simulink model "automata"  (R2020b)
settings: Solver=VariableStepAuto  StartTime=0.0  StopTime=100  RelTol=1e-3
model workspace (MAT data in the model file):
  G_sup_tsp = Simulink.Signal
  G_sup_tsp.DataType = 'double'
  G_sup_tsp.Dimensions = -1
  G_sup_tsp.DimensionsMode = 'auto'
  G_sup_tsp.Complexity = 'real'
  G_sup_tsp.SampleTime = -1
  G_sup_tsp.SamplingMode = 'auto'
  G_sup_tsp.InitialValue = '175'
  G_sup_tsp_ideal = Simulink.Signal
  G_sup_tsp_ideal.DataType = 'double'
  G_sup_tsp_ideal.Dimensions = -1
  G_sup_tsp_ideal.DimensionsMode = 'auto'
  G_sup_tsp_ideal.Complexity = 'real'
  G_sup_tsp_ideal.SampleTime = -1
  G_sup_tsp_ideal.SamplingMode = 'auto'
  G_sup_tsp_ideal.InitialValue = '175'
  G_sup_tsp_noneAct = Simulink.Signal
  G_sup_tsp_noneAct.DataType = 'double'
  G_sup_tsp_noneAct.Dimensions = -1
  G_sup_tsp_noneAct.DimensionsMode = 'auto'
  G_sup_tsp_noneAct.Complexity = 'real'
  G_sup_tsp_noneAct.SampleTime = -1
  G_sup_tsp_noneAct.SamplingMode = 'auto'
  G_sup_tsp_noneAct.InitialValue = '175'
undefined symbols (not defined in the file): WLAN
libraries: truetime x3, pid_lib x2, simulink x1
settings Model: Creator=Mr_Li  LastModifiedBy=Mr_Li

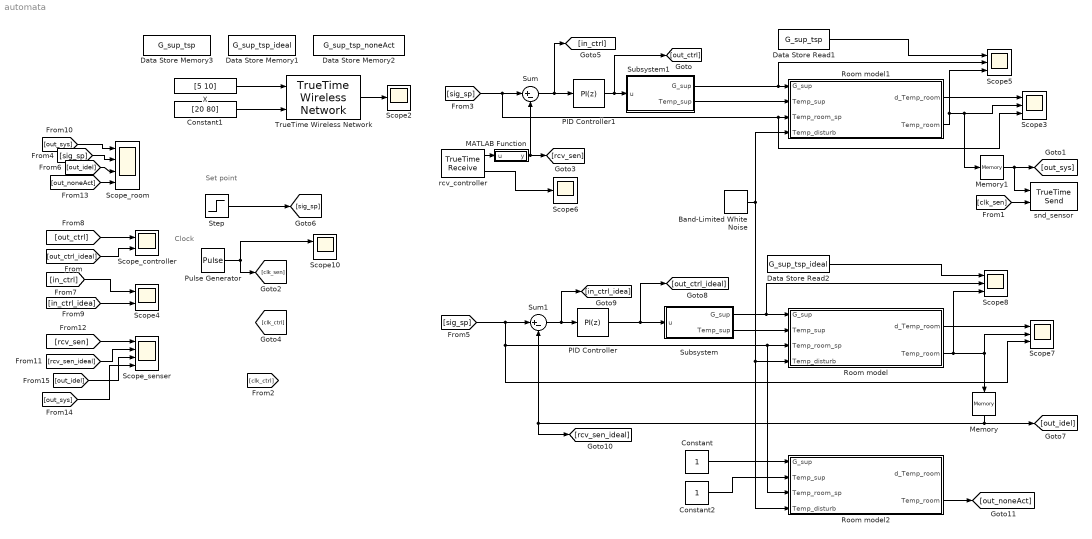
== system automata ==
  note: Set point
  note: Clock
  Band-Limited White Noise : simulink/Sources/Band-Limited White Noise  Cov=[0.01]  Ts=1  seed=[23341]
  Constant : Constant
  Constant1 : Constant  Value=[20 80]  VectorParams1D=off
  Constant2 : Constant
  Data Store Memory1 : DataStoreMemory  DataStoreName=G_sup_tsp_ideal  ReadBeforeWriteMsg=warning  WriteAfterWriteMsg=warning  WriteAfterReadMsg=warning  InitialValue=175  ShowAdditionalParam=off  OutDataTypeStr=double
  Data Store Memory2 : DataStoreMemory  DataStoreName=G_sup_tsp_noneAct  ReadBeforeWriteMsg=warning  WriteAfterWriteMsg=warning  WriteAfterReadMsg=warning  InitialValue=175  ShowAdditionalParam=off  OutDataTypeStr=double
  Data Store Memory3 : DataStoreMemory  DataStoreName=G_sup_tsp  ReadBeforeWriteMsg=warning  WriteAfterWriteMsg=warning  WriteAfterReadMsg=warning  InitialValue=175  ShowAdditionalParam=off  OutDataTypeStr=double
  Data Store Read1 : DataStoreRead  DataStoreName=G_sup_tsp
  Data Store Read2 : DataStoreRead  DataStoreName=G_sup_tsp_ideal
  MATLAB Function : MATLAB Function  TreatAsAtomicUnit=on
  Memory : Memory  InitialCondition=21
  Memory1 : Memory  InitialCondition=21
  PID Controller : pid_lib/PID Controller  Controller=PI  Form=Parallel  TimeDomain=Discrete-time  UseExternalTs=off  SampleTime=5  IntegratorMethod=Forward Euler  FilterMethod=Forward Euler  ControllerParametersSource=internal  P=350  I=15  D=0  UseFilter=on  N=100  TunerSelectOption=Transfer Function Based (PID Tuner App)  InitialConditionSource=internal  InitialConditionForIntegrator=0  InitialConditionForFilter=0  DifferentiatorICPrevScaledInput=0  ExternalReset=none  TrackingMode=off  Kt=1  LimitOutput=on  SatLimitsSource=internal  UpperSaturationLimit=2000  LowerSaturationLimit=100  LinearizeAsGain=on  AntiWindupMode=none  Kb=1  POutMin=[]  POutMax=[]  IOutMin=[]  IOutMax=[]  DOutMin=[]  DOutMax=[]  NOutMin=[]  NOutMax=[]  SumOutMin=[]  SumOutMax=[]  SaturationOutMin=[]  SaturationOutMax=[]  PParamMin=[]  PParamMax=[]  IParamMin=[]  IParamMax=[]  DParamMin=[]  DParamMax=[]  NParamMin=[]  NParamMax=[]  KbParamMin=[]  KbParamMax=[]  KtParamMin=[]  KtParamMax=[]  KbOutMin=[]  KbOutMax=[]  KtOutMin=[]  KtOutMax=[]  IntegratorOutMin=[]  IntegratorOutMax=[]  FilterOutMin=[]  FilterOutMax=[]  SumI1OutMin=[]  SumI1OutMax=[]  SumI2OutMin=[]  SumI2OutMax=[]  SumI3OutMin=[]  SumI3OutMax=[]  SumI4OutMin=[]  SumI4OutMax=[]  SumDOutMin=[]  SumDOutMax=[]  DifferentiatorOutMin=[]  DifferentiatorOutMax=[]  FilterDiffOutCoefMin=[]  FilterDiffOutCoefMax=[]  ReciprocalOutMin=[]  ReciprocalOutMax=[]  SumDenOutMin=[]  SumDenOutMax=[]  SumNumOutMin=[]  SumNumOutMax=[]  DivideOutMin=[]  DivideOutMax=[]  UdiffTsProdOutMin=[]  UdiffTsProdOutMax=[]  NTsProdOutMin=[]  NTsProdOutMax=[]  UintegralTsProdOutMin=[]  UintegralTsProdOutMax=[]  UngainTsProdOutMin=[]  UngainTsProdOutMax=[]  IntegratorContinuousStateAttributes=''  IntegratorStateMustResolveToSignalObject=off  IntegratorRTWStateStorageClass=Auto  FilterContinuousStateAttributes=''  FilterStateMustResolveToSignalObject=off  FilterRTWStateStorageClass=Auto  ParallelPVariant=InternalParameters  IdealPVariant=Disabled  IVariant=InternalParameters  DVariant=Disabled  IntegratorVariant=Discrete  SatVariant=Enabled  AWVariant=Passthrough  PCopyVariant=Disabled  TRVariant=Disabled  FdbkBlocksVariant=Forward  IdealPFdbkVariant=Disabled  SatFdbkVariant=Disabled  DerivativeFilterVariant=Disabled  NVariant=Disabled  NCopyVariant=Disabled_SignalSpec  FilterICVariant=Disabled  IntegratorICVariant=InternalICs  ExternalResetVariant=Disabled  TRSumVariant=Passthrough  SumFdbkVariant=Disabled  SumVariant=Sum_PI  TsampFilterVariant=InternalTs  TsampNgainVariant=Passthrough  TsampIntegralVariant=Passthrough  ExternalSaturationOutDataTypeStr=Inherit: Same as second input
  PID Controller1 : pid_lib/PID Controller  Controller=PI  Form=Parallel  TimeDomain=Discrete-time  UseExternalTs=off  SampleTime=5  IntegratorMethod=Forward Euler  FilterMethod=Forward Euler  ControllerParametersSource=internal  P=350  I=15  D=0  UseFilter=on  N=100  TunerSelectOption=Transfer Function Based (PID Tuner App)  InitialConditionSource=internal  InitialConditionForIntegrator=0  InitialConditionForFilter=0  DifferentiatorICPrevScaledInput=0  ExternalReset=none  TrackingMode=off  Kt=1  LimitOutput=on  SatLimitsSource=internal  UpperSaturationLimit=2000  LowerSaturationLimit=100  LinearizeAsGain=on  AntiWindupMode=none  Kb=1  POutMin=[]  POutMax=[]  IOutMin=[]  IOutMax=[]  DOutMin=[]  DOutMax=[]  NOutMin=[]  NOutMax=[]  SumOutMin=[]  SumOutMax=[]  SaturationOutMin=[]  SaturationOutMax=[]  PParamMin=[]  PParamMax=[]  IParamMin=[]  IParamMax=[]  DParamMin=[]  DParamMax=[]  NParamMin=[]  NParamMax=[]  KbParamMin=[]  KbParamMax=[]  KtParamMin=[]  KtParamMax=[]  KbOutMin=[]  KbOutMax=[]  KtOutMin=[]  KtOutMax=[]  IntegratorOutMin=[]  IntegratorOutMax=[]  FilterOutMin=[]  FilterOutMax=[]  SumI1OutMin=[]  SumI1OutMax=[]  SumI2OutMin=[]  SumI2OutMax=[]  SumI3OutMin=[]  SumI3OutMax=[]  SumI4OutMin=[]  SumI4OutMax=[]  SumDOutMin=[]  SumDOutMax=[]  DifferentiatorOutMin=[]  DifferentiatorOutMax=[]  FilterDiffOutCoefMin=[]  FilterDiffOutCoefMax=[]  ReciprocalOutMin=[]  ReciprocalOutMax=[]  SumDenOutMin=[]  SumDenOutMax=[]  SumNumOutMin=[]  SumNumOutMax=[]  DivideOutMin=[]  DivideOutMax=[]  UdiffTsProdOutMin=[]  UdiffTsProdOutMax=[]  NTsProdOutMin=[]  NTsProdOutMax=[]  UintegralTsProdOutMin=[]  UintegralTsProdOutMax=[]  UngainTsProdOutMin=[]  UngainTsProdOutMax=[]  IntegratorContinuousStateAttributes=''  IntegratorStateMustResolveToSignalObject=off  IntegratorRTWStateStorageClass=Auto  FilterContinuousStateAttributes=''  FilterStateMustResolveToSignalObject=off  FilterRTWStateStorageClass=Auto  ParallelPVariant=InternalParameters  IdealPVariant=Disabled  IVariant=InternalParameters  DVariant=Disabled  IntegratorVariant=Discrete  SatVariant=Enabled  AWVariant=Passthrough  PCopyVariant=Disabled  TRVariant=Disabled  FdbkBlocksVariant=Forward  IdealPFdbkVariant=Disabled  SatFdbkVariant=Disabled  DerivativeFilterVariant=Disabled  NVariant=Disabled  NCopyVariant=Disabled_SignalSpec  FilterICVariant=Disabled  IntegratorICVariant=InternalICs  ExternalResetVariant=Disabled  TRSumVariant=Passthrough  SumFdbkVariant=Disabled  SumVariant=Sum_PI  TsampFilterVariant=InternalTs  TsampNgainVariant=Passthrough  TsampIntegralVariant=Passthrough  ExternalSaturationOutDataTypeStr=Inherit: Same as second input
  Pulse Generator : DiscretePulseGenerator  Period=5
  Room model : Subsystem  mask{a0=5.71, a1=-0.099, a2=-0.0004, a3=-0.25, V_r=50, gamma=0.9, StableThreshold=0.5}
      mask prompts: StableThreshold "Set stable threshold of indoor temperature"
  Room model1 : Subsystem  mask{a0=5.71, a1=-0.099, a2=-0.0004, a3=-0.25, V_r=50, gamma=0.9, StableThreshold=0.5}
      mask prompts: StableThreshold "Set stable threshold of indoor temperature"
  Room model2 : Subsystem  mask{a0=5.71, a1=-0.099, a2=-0.0004, a3=-0.25, V_r=50, gamma=0.9, StableThreshold=0.5}
      mask prompts: StableThreshold "Set stable threshold of indoor temperature"
  Scope10 : Scope  NumInputPorts=2
  Scope2 : Scope
  Scope{3,5,7..8} (4 alike) : Scope  NumInputPorts=3
  Scope4 : Scope  NumInputPorts=2
  Scope6 : Scope
  Scope_controller : Scope  NumInputPorts=2
  Scope_room : Scope  NumInputPorts=4
  Scope_senser : Scope  NumInputPorts=4
  Step : Step  Time=5  Before=23  After=23
  Subsystem : Subsystem
  Subsystem1 : Subsystem
  Sum : Sum  Inputs=|+-
  Sum1 : Sum  Inputs=|+-
  TrueTime Wireless Network : truetime/TrueTime Wireless  Network  nwtype=802.11b (WLAN)  nwnbr=1  nnodes=2  rate=800000  minsize=272  transpower=30  threshold=-48  use_pathloss_function=default  pathloss=4.0  acktimeout=1  retrylimit=3  error_threshold=0.04  lossprob=0.3  seed=0  scheduleoutput=on  poweroutput=off
  X : Constant  Value=[5 10]  VectorParams1D=off
  rcv_controller : truetime/TrueTime Receive  nwnbr=1  receiver=2  outdim=1  triggeroutput=on  senderoutput=off  lengthoutput=off  priorityoutput=off  timestampoutput=off  signalpoweroutput=off  msgIDoutput=off
  snd_sensor : truetime/TrueTime Send  trigger=falling  nwnbr=1  sender=1  indim=1  recsource=internal  receiver=2  lengthsource=internal  length=1000  priosource=internal  prio=1  msgIDsource=internal  msgID=0  dynamicSegment=dynamic
  wires:
  Sum1/1 -> PID Controller/1, [in_ctrl_idea]
  PID Controller/1 -> Subsystem/1(u), [out_ctrl_ideal]
  [sig_sp] -> Scope7/3, Room model2/3(Temp_room_sp), Room model/3(Temp_room_sp), Sum1/1
  Room model/1(d_Temp_room) -> Scope7/1
  Memory/1 -> Sum1/2, [rcv_sen_ideal], [out_idel]
  Room model/2(Temp_room) -> Scope8/3, Scope7/2, Memory/1
  Subsystem/2(Temp_sup) -> Room model/2(Temp_sup)
  Subsystem/1(G_sup) -> Room model/1(G_sup), Scope8/2
  Data Store Read2/1 -> Scope8/1
  X/1 -> TrueTime Wireless Network/1
  Constant1/1 -> TrueTime Wireless Network/2
  TrueTime Wireless Network/1 -> Scope2/1
  Memory1/1 -> [out_sys], snd_sensor/1
  rcv_controller/2 -> Scope6/1
  Step/1 -> [sig_sp]
  [sig_sp] -> Scope_room/2
  [out_idel] -> Scope_room/3
  [out_sys] -> Scope_room/1
  [in_ctrl_idea] -> Scope4/2
  [out_ctrl] -> Scope_controller/1
  [out_ctrl_ideal] -> Scope_controller/2
  [in_ctrl] -> Scope4/1
  Sum/1 -> [in_ctrl], PID Controller1/1
  Room model1/2(Temp_room) -> Scope5/3, Scope3/2, Memory1/1
  Subsystem1/2(Temp_sup) -> Room model1/2(Temp_sup)
  Subsystem1/1(G_sup) -> Scope5/2, Room model1/1(G_sup)
  PID Controller1/1 -> [out_ctrl], Subsystem1/1(u)
  Room model1/1(d_Temp_room) -> Scope3/1
  Data Store Read1/1 -> Scope5/1
  [sig_sp] -> Scope3/3, Room model1/3(Temp_room_sp), Sum/1
  Band-Limited White Noise/1 -> Room model2/4(Temp_disturb), Room model/4(Temp_disturb), Room model1/4(Temp_disturb)
  [rcv_sen] -> Scope_senser/1
  [rcv_sen_ideal] -> Scope_senser/2
  Pulse Generator/1 -> [clk_sen], Scope10/1
  [clk_sen] -> snd_sensor/2
  rcv_controller/1 -> MATLAB Function/1(u)
  MATLAB Function/1(y) -> Sum/2, [rcv_sen]
  Constant/1 -> Room model2/1(G_sup)
  Constant2/1 -> Room model2/2(Temp_sup)
  Room model2/2(Temp_room) -> [out_noneAct]
  [out_noneAct] -> Scope_room/4
  [out_idel] -> Scope_senser/3
  [out_sys] -> Scope_senser/4

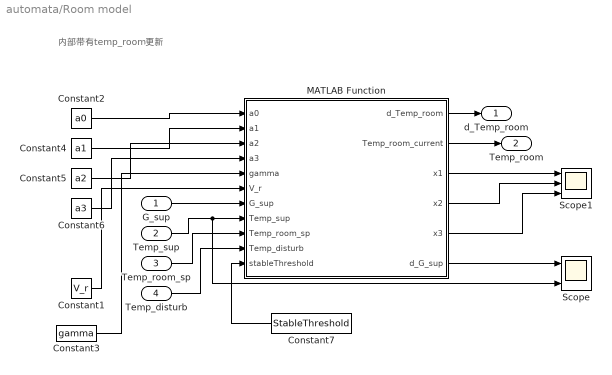
== system automata/Room model ==
  note: 内部带有temp_room更新
  G_sup : Inport
  Temp_sup : Inport  Port=2
  Temp_room_sp : Inport  Port=3
  Temp_disturb : Inport  Port=4
  Constant1 : Constant  Value=V_r
  Constant2 : Constant  Value=a0
  Constant3 : Constant  Value=gamma
  Constant4 : Constant  Value=a1
  Constant5 : Constant  Value=a2
  Constant6 : Constant  Value=a3
  Constant7 : Constant  Value=StableThreshold
  MATLAB Function : MATLAB Function  TreatAsAtomicUnit=on
  Scope : Scope  NumInputPorts=3
  Scope1 : Scope  NumInputPorts=3
  d_Temp_room : Outport
  Temp_room : Outport  Port=2
  wires:
  MATLAB Function/1(d_Temp_room) -> d_Temp_room/1
  Temp_sup/1 -> Scope/3, MATLAB Function/8(Temp_sup)
  MATLAB Function/4(x2) -> Scope1/2
  Constant2/1 -> MATLAB Function/1(a0)
  G_sup/1 -> MATLAB Function/7(G_sup)
  Constant1/1 -> MATLAB Function/6(V_r)
  Constant3/1 -> MATLAB Function/5(gamma)
  Constant6/1 -> MATLAB Function/4(a3)
  Constant5/1 -> MATLAB Function/3(a2)
  Temp_room_sp/1 -> MATLAB Function/9(Temp_room_sp)
  Constant4/1 -> MATLAB Function/2(a1)
  MATLAB Function/3(x1) -> Scope1/1
  MATLAB Function/2(Temp_room_current) -> Temp_room/1
  Constant7/1 -> MATLAB Function/11(stableThreshold)
  MATLAB Function/6(d_G_sup) -> Scope/1
  MATLAB Function/5(x3) -> Scope1/3
  Temp_disturb/1 -> MATLAB Function/10(Temp_disturb)

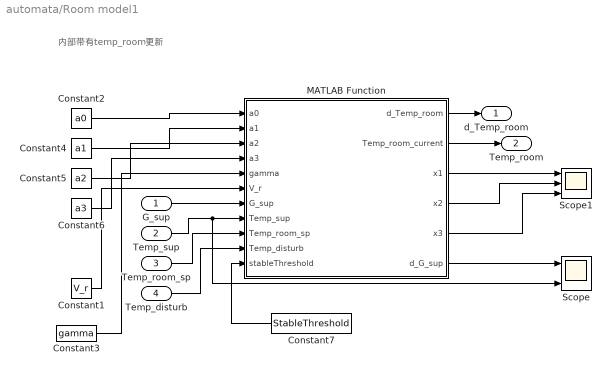
== system automata/Room model1 ==
  note: 内部带有temp_room更新
  G_sup : Inport
  Temp_sup : Inport  Port=2
  Temp_room_sp : Inport  Port=3
  Temp_disturb : Inport  Port=4
  Constant1 : Constant  Value=V_r
  Constant2 : Constant  Value=a0
  Constant3 : Constant  Value=gamma
  Constant4 : Constant  Value=a1
  Constant5 : Constant  Value=a2
  Constant6 : Constant  Value=a3
  Constant7 : Constant  Value=StableThreshold
  MATLAB Function : MATLAB Function  TreatAsAtomicUnit=on
  Scope : Scope  NumInputPorts=3
  Scope1 : Scope  NumInputPorts=3
  d_Temp_room : Outport
  Temp_room : Outport  Port=2
  wires:
  MATLAB Function/1(d_Temp_room) -> d_Temp_room/1
  Temp_sup/1 -> Scope/3, MATLAB Function/8(Temp_sup)
  MATLAB Function/4(x2) -> Scope1/2
  Constant2/1 -> MATLAB Function/1(a0)
  G_sup/1 -> MATLAB Function/7(G_sup)
  Constant1/1 -> MATLAB Function/6(V_r)
  Constant3/1 -> MATLAB Function/5(gamma)
  Constant6/1 -> MATLAB Function/4(a3)
  Constant5/1 -> MATLAB Function/3(a2)
  Temp_room_sp/1 -> MATLAB Function/9(Temp_room_sp)
  Constant4/1 -> MATLAB Function/2(a1)
  MATLAB Function/3(x1) -> Scope1/1
  MATLAB Function/2(Temp_room_current) -> Temp_room/1
  Constant7/1 -> MATLAB Function/11(stableThreshold)
  MATLAB Function/6(d_G_sup) -> Scope/1
  MATLAB Function/5(x3) -> Scope1/3
  Temp_disturb/1 -> MATLAB Function/10(Temp_disturb)

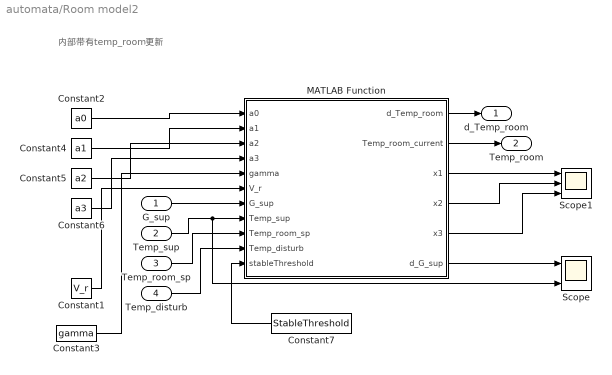
== system automata/Room model2 ==
  note: 内部带有temp_room更新
  G_sup : Inport
  Temp_sup : Inport  Port=2
  Temp_room_sp : Inport  Port=3
  Temp_disturb : Inport  Port=4
  Constant1 : Constant  Value=V_r
  Constant2 : Constant  Value=a0
  Constant3 : Constant  Value=gamma
  Constant4 : Constant  Value=a1
  Constant5 : Constant  Value=a2
  Constant6 : Constant  Value=a3
  Constant7 : Constant  Value=StableThreshold
  MATLAB Function : MATLAB Function  TreatAsAtomicUnit=on
  Scope : Scope  NumInputPorts=3
  Scope1 : Scope  NumInputPorts=3
  d_Temp_room : Outport
  Temp_room : Outport  Port=2
  wires:
  MATLAB Function/1(d_Temp_room) -> d_Temp_room/1
  Temp_sup/1 -> Scope/3, MATLAB Function/8(Temp_sup)
  MATLAB Function/4(x2) -> Scope1/2
  Constant2/1 -> MATLAB Function/1(a0)
  G_sup/1 -> MATLAB Function/7(G_sup)
  Constant1/1 -> MATLAB Function/6(V_r)
  Constant3/1 -> MATLAB Function/5(gamma)
  Constant6/1 -> MATLAB Function/4(a3)
  Constant5/1 -> MATLAB Function/3(a2)
  Temp_room_sp/1 -> MATLAB Function/9(Temp_room_sp)
  Constant4/1 -> MATLAB Function/2(a1)
  MATLAB Function/3(x1) -> Scope1/1
  MATLAB Function/2(Temp_room_current) -> Temp_room/1
  Constant7/1 -> MATLAB Function/11(stableThreshold)
  MATLAB Function/6(d_G_sup) -> Scope/1
  MATLAB Function/5(x3) -> Scope1/3
  Temp_disturb/1 -> MATLAB Function/10(Temp_disturb)

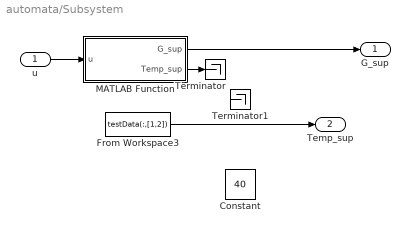
== system automata/Subsystem ==
  u : Inport
  Constant : Constant  Value=40
  From Workspace3 : FromWorkspace  VariableName=testData(:,[1,2])  SampleTime=1
  MATLAB Function : MATLAB Function  TreatAsAtomicUnit=on
  Terminator : Terminator
  Terminator1 : Terminator
  G_sup : Outport
  Temp_sup : Outport  Port=2
  wires:
  u/1 -> MATLAB Function/1(u)
  MATLAB Function/1(G_sup) -> G_sup/1
  MATLAB Function/2(Temp_sup) -> Terminator/1
  From Workspace3/1 -> Temp_sup/1

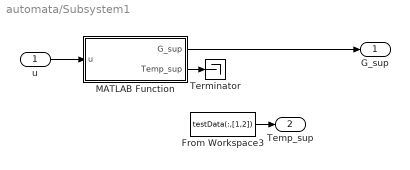
== system automata/Subsystem1 ==
  u : Inport
  From Workspace3 : FromWorkspace  VariableName=testData(:,[1,2])  SampleTime=1
  MATLAB Function : MATLAB Function  TreatAsAtomicUnit=on
  Terminator : Terminator
  G_sup : Outport
  Temp_sup : Outport  Port=2
  wires:
  u/1 -> MATLAB Function/1(u)
  MATLAB Function/1(G_sup) -> G_sup/1
  From Workspace3/1 -> Temp_sup/1
  MATLAB Function/2(Temp_sup) -> Terminator/1

== matlab function automata/Subsystem/MATLAB Function ==
  data: u input; G_sup output; Temp_sup output
function [G_sup,Temp_sup] = fcn(u)

persistent G;
if(isempty(G))
    G=800;
end


d_G_sup=u-G;
G_sup=u;
G=u;

Temp_sup=40;

== matlab function automata/Room model1/MATLAB Function ==
  settings: updateMethod=DISCRETE  sampleTime=1
  data: a0 input; d_Temp_room output; Temp_room_current output; a1 input; a2 input; a3 input; gamma input; V_r input; G_sup input; Temp_sup input; Temp_room_sp input; Temp_disturb input; stableThreshold input; x1 output; x2 output; x3 output; G_sup_tsp data_store_memory; d_G_sup output

function [d_Temp_room,Temp_room_current,x1,x2,x3,d_G_sup] = fcn(a0,a1,a2,a3,gamma,V_r,G_sup,Temp_sup,Temp_room_sp,Temp_disturb,stableThreshold)

persistent Temp_room_buffer;
persistent BufferCount;
persistent Temp_room;
persistent G;
global G_sup_tsp;

% 对静态变量初始化
if(isempty(Temp_room_buffer))
   Temp_room_buffer= [22.1000   21.8000   21.5000   21.2000   21.0000];
end

if(isempty(Temp_room))
    Temp_room=21;
end

if(isempty(BufferCount))
    BufferCount=0;
end

if(isempty(G))
    G=310;
end
    
d_G_sup=G_sup-G;

% 室内温度存储缓冲器，即选取前n=5时刻的室内温度
% 思路：根据BufferCount进行取模，轮流更替index，从n=5数组中选取变量
Temp_room_5prev=Temp_room_buffer(mod(BufferCount,5)+1);


% 计算a,b参数值
a = gamma*G_sup_tsp/V_r;
b = (Temp_sup-(gamma*Temp_room_sp))*d_G_sup/V_r;

x1=(-1)*(b/a)*exp(-1*a);
x2=(b/a);
x3=Temp_room_5prev;

d_Temp_room = a0+ a1*x1+ a2*x2+ a3*Temp_room_5prev;

Temp_room=Temp_room+d_Temp_room+Temp_disturb;
Temp_room_current=Temp_room;
Temp_room_buffer(mod(BufferCount,5)+1)=Temp_room;

BufferCount=BufferCount+1;

G=G_sup;


% 更新G_sup_tsp
if(abs(Temp_room-Temp_room_sp)<stableThreshold)
        G_sup_tsp=G_sup;
else
     G_sup_tsp=G_sup_tsp;
end


end

== matlab function automata/Room model/MATLAB Function ==
  settings: updateMethod=DISCRETE  sampleTime=1
  data: a0 input; d_Temp_room output; Temp_room_current output; a1 input; a2 input; a3 input; gamma input; V_r input; G_sup input; Temp_sup input; Temp_room_sp input; Temp_disturb input; stableThreshold input; x1 output; x2 output; x3 output; G_sup_tsp_ideal data_store_memory; d_G_sup output

function [d_Temp_room,Temp_room_current,x1,x2,x3,d_G_sup] = fcn(a0,a1,a2,a3,gamma,V_r,G_sup,Temp_sup,Temp_room_sp,Temp_disturb,stableThreshold)

persistent Temp_room_buffer;
persistent BufferCount;
persistent Temp_room;
persistent G;
global G_sup_tsp_ideal;

% 对静态变量初始化
if(isempty(Temp_room_buffer))
   Temp_room_buffer= [22.1000   21.8000   21.5000   21.2000   21.0000];
end

if(isempty(Temp_room))
    Temp_room=21;
end

if(isempty(BufferCount))
    BufferCount=0;
end

if(isempty(G))
    G=310;
end
    
d_G_sup=G_sup-G;

% 室内温度存储缓冲器，即选取前n=5时刻的室内温度
% 思路：根据BufferCount进行取模，轮流更替index，从n=5数组中选取变量
Temp_room_5prev=Temp_room_buffer(mod(BufferCount,5)+1);


% 计算a,b参数值
a = gamma*G_sup_tsp_ideal/V_r;
b = (Temp_sup-(gamma*Temp_room_sp))*d_G_sup/V_r;

x1=(-1)*(b/a)*exp(-1*a);
x2=(b/a);
x3=Temp_room_5prev;

d_Temp_room = a0+ a1*x1+ a2*x2+ a3*Temp_room_5prev;

Temp_room=Temp_room+d_Temp_room+Temp_disturb;
Temp_room_current=Temp_room;
Temp_room_buffer(mod(BufferCount,5)+1)=Temp_room;

BufferCount=BufferCount+1;

G=G_sup;


% 更新G_sup_tsp
if(abs(Temp_room-Temp_room_sp)<stableThreshold)
        G_sup_tsp_ideal=G_sup;
else
     G_sup_tsp_ideal=G_sup_tsp_ideal;
end


end

== matlab function automata/Subsystem1/MATLAB Function ==
  data: u input; G_sup output; Temp_sup output
function [G_sup,Temp_sup] = fcn(u)

persistent G;
if(isempty(G))
    G=800;
end


d_G_sup=u-G;
G_sup=u;
G=u;

Temp_sup=40;

== matlab function automata/MATLAB Function ==
  data: u input; y output
function y = initialHolder(u)
persistent u0;
if(isempty(u0))
    u0=21;
end

if(u==0)
    y=u0;
else
    y = u;
    u0=u;
end

== matlab function automata/Room model2/MATLAB Function ==
  settings: updateMethod=DISCRETE  sampleTime=1
  data: a0 input; d_Temp_room output; Temp_room_current output; a1 input; a2 input; a3 input; gamma input; V_r input; G_sup input; Temp_sup input; Temp_room_sp input; Temp_disturb input; stableThreshold input; x1 output; x2 output; x3 output; G_sup_tsp_noneAct data_store_memory; d_G_sup output

function [d_Temp_room,Temp_room_current,x1,x2,x3,d_G_sup] = fcn(a0,a1,a2,a3,gamma,V_r,G_sup,Temp_sup,Temp_room_sp,Temp_disturb,stableThreshold)

persistent Temp_room_buffer;
persistent BufferCount;
persistent Temp_room;
persistent G;
global G_sup_tsp_noneAct;

% 对静态变量初始化
if(isempty(Temp_room_buffer))
   Temp_room_buffer= [22.1000   21.8000   21.5000   21.2000   21.0000];
end

if(isempty(Temp_room))
    Temp_room=21;
end

if(isempty(BufferCount))
    BufferCount=0;
end

if(isempty(G))
    G=310;
end
    
d_G_sup=G_sup-G;

% 室内温度存储缓冲器，即选取前n=5时刻的室内温度
% 思路：根据BufferCount进行取模，轮流更替index，从n=5数组中选取变量
Temp_room_5prev=Temp_room_buffer(mod(BufferCount,5)+1);


% 计算a,b参数值
a = gamma*G_sup_tsp_noneAct/V_r;
b = (Temp_sup-(gamma*Temp_room_sp))*d_G_sup/V_r;

x1=(-1)*(b/a)*exp(-1*a);
x2=(b/a);
x3=Temp_room_5prev;

d_Temp_room = a0+ a1*x1+ a2*x2+ a3*Temp_room_5prev;

Temp_room=Temp_room+d_Temp_room+Temp_disturb;
Temp_room_current=Temp_room;
Temp_room_buffer(mod(BufferCount,5)+1)=Temp_room;

BufferCount=BufferCount+1;

G=G_sup;


% 更新G_sup_tsp
if(abs(Temp_room-Temp_room_sp)<stableThreshold)
        G_sup_tsp_noneAct=G_sup;
else
     G_sup_tsp_noneAct=G_sup_tsp_noneAct;
end


end
